simulink model "lookupTableDynamic_TestGen20"  (R2017b)
settings: Solver=FixedStepDiscrete  StartTime=0.0  StopTime=10.0  RelTol=1e-3
libraries: simulink x1
settings Model: Creator=ktrinh  LastModifiedBy=ktrinh
settings DebuggingCC: ParameterOverflowMsg=none

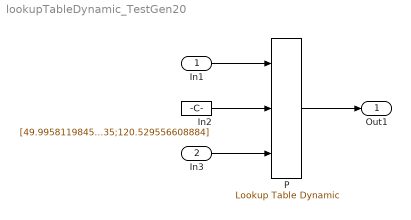
== system lookupTableDynamic_TestGen20 ==
  In1 : Inport  OutMin=47.9958  OutMax=123  OutDataTypeStr=uint8  PortDimensions=1
  In3 : Inport  Port=2  PortDimensions=5
  In2 : Constant  Value=[49.9958119845767;63.435920185164;93.1596889776251;119.33030578135;120.529556608884]  OutDataTypeStr=uint8
  P : simulink/Lookup Tables/Lookup Table Dynamic  LookUpMeth=Use Input Nearest  OutDataType=fixdt('single')  OutScaling=[]  OutputDataTypeScalingMode=Specify via dialog  OutDataTypeStr=single  RndMeth=Zero  DoSatur=off
      settings: SourceProductName=Simulink
  Out1 : Outport
  wires:
  In1/1 -> P/1
  In2/1 -> P/2
  In3/1 -> P/3
  P/1 -> Out1/1
